simulink model "RoundDemo"  (Simulink 6.3)
settings: Solver=FixedStepDiscrete  StartTime=0.0  StopTime=10.0  FixedStep=1  RelTol=1e-3
InitFcn:
  | %% DSPBuilder Start
  | alt_dspbuilder_update_model(bdroot)
  | %% DSPBuilder End
libraries: allblocks_alteradspbuilder2 x7
settings Model: LastModifiedBy=delphick

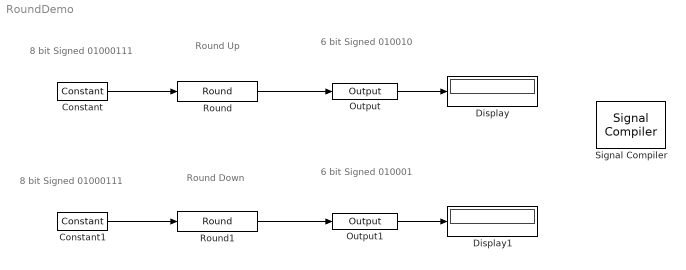
== system RoundDemo ==
  note: 8 bit Signed
      | 01000111
  note: 6 bit Signed
      | 010010
  note: Round Up
  note: Round Down
  note: 8 bit Signed
      | 01000111
  note: 6 bit Signed
      | 010001
  Constant : allblocks_alteradspbuilder2/Constant  mask_cst=71  BusType=Signed Integer  bwl=8  bwr=0  SpecifyClock=off
  Constant1 : allblocks_alteradspbuilder2/Constant  mask_cst=71  BusType=Signed Integer  bwl=8  bwr=0  SpecifyClock=off
  Display : Display
  Display1 : Display
  Output : allblocks_alteradspbuilder2/Output  iofile=C:\workspace_clean\Documentation\DesignExamples\Tutorials\UnitBlocks\IOBus\Round\tb_RoundDemo\RoundDemo_Output.capture  BusType=Signed Integer  bwl=6  bwr=0  PORTTYPE=Output
  Output1 : allblocks_alteradspbuilder2/Output  iofile=C:\workspace_clean\Documentation\DesignExamples\Tutorials\UnitBlocks\IOBus\Round\tb_RoundDemo\RoundDemo_Output1.capture  BusType=Signed Integer  bwl=6  bwr=0  PORTTYPE=Output
  Round : allblocks_alteradspbuilder2/Round  BusType=Signed Integer  bwl=8  bwr=1  bitsToRemove=2  roundMode=ROUND_UP  userRoundMode=Round To Plus Infinity  pipeline=off
  Round1 : allblocks_alteradspbuilder2/Round  BusType=Signed Integer  bwl=8  bwr=1  bitsToRemove=2  roundMode=TRUNCATE_LOW  userRoundMode=Truncate  pipeline=off
  Signal Compiler : allblocks_alteradspbuilder2/Signal Compiler  DeviceFamily=Stratix IV  DeviceName=AUTO  EnableSignalTap=off  SignalTapDepth=128  UseBoardBlock=off  StpUseDefaultClock=on  StpClock=clock
  wires:
  Constant/1 -> Round/1
  Round/1 -> Output/1
  Output/1 -> Display/1
  Constant1/1 -> Round1/1
  Round1/1 -> Output1/1
  Output1/1 -> Display1/1
